simulink model "Extended_2"  (R2019a)
settings: Solver=VariableStepAuto  StartTime=0.0  StopTime=5  RelTol=1e-3
values from neighbouring files (symbols this model uses):
  g = 9.81    [Data.m]    (also in func.m; myTransitionFcn.m)
  m = 0.1    [Data.m]    (also in myTransitionFcn.m)
  r = 0.1    [Data.m]    (also in func.m; myTransitionFcn.m)
  R = 1    [Data.m]    (also in func.m; myTransitionFcn.m)
libraries: simulink x3
settings Model: Creator=Dell  LastModifiedBy=Dell

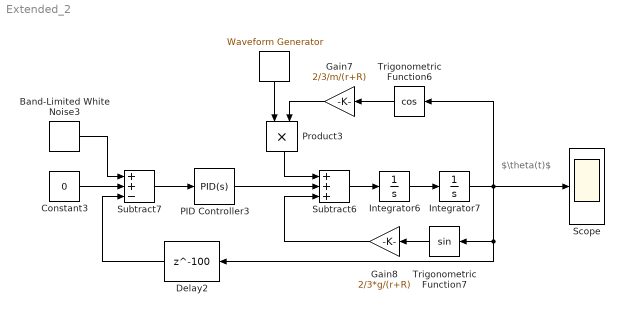
== system Extended_2 ==
  note: $\theta(t)$
  " " : simulink/Sources/Waveform Generator  OutMin=[]  OutMax=[]  OutDataTypeStr=double  SelectedSignal=1  Signals=step()  BlockNames=MultiportSwitch_8c7b78d12e5b405  SampleTime=0.1
      settings: SourceProductName=Simulink
  Band-Limited White Noise3 : simulink/Sources/Band-Limited White Noise  Cov=[0.0001]  Ts=0.1  seed=[23341]
  Constant3 : Constant  Value=0
  Delay2 : Delay  DelayLength=100  InitialCondition=0  UseCircularBuffer=on
  Gain7 : Gain  Gain=2/3/m/(r+R)
  Gain8 : Gain  Gain=2/3*g/(r+R)
  Integrator6 : Integrator
  Integrator7 : Integrator
  PID Controller3 : simulink/Continuous/PID Controller  Controller=PID  Form=Parallel  TimeDomain=Continuous-time  SampleTime=-1  IntegratorMethod=Forward Euler  FilterMethod=Forward Euler  ControllerParametersSource=internal  P=11  I=10  D=6  UseFilter=on  N=141.793807285204  TunerSelectOption=Transfer Function Based (PID Tuner App)  InitialConditionSource=internal  InitialConditionForIntegrator=0  InitialConditionForFilter=0  DifferentiatorICPrevScaledInput=0  ExternalReset=none  TrackingMode=off  Kt=1  LimitOutput=off  UpperSaturationLimit=inf  LowerSaturationLimit=-inf  LinearizeAsGain=on  AntiWindupMode=none  Kb=1  POutMin=[]  POutMax=[]  IOutMin=[]  IOutMax=[]  DOutMin=[]  DOutMax=[]  NOutMin=[]  NOutMax=[]  SumOutMin=[]  SumOutMax=[]  SaturationOutMin=[]  SaturationOutMax=[]  PParamMin=[]  PParamMax=[]  IParamMin=[]  IParamMax=[]  DParamMin=[]  DParamMax=[]  NParamMin=[]  NParamMax=[]  KbParamMin=[]  KbParamMax=[]  KtParamMin=[]  KtParamMax=[]  KbOutMin=[]  KbOutMax=[]  KtOutMin=[]  KtOutMax=[]  IntegratorOutMin=[]  IntegratorOutMax=[]  FilterOutMin=[]  FilterOutMax=[]  SumI1OutMin=[]  SumI1OutMax=[]  SumI2OutMin=[]  SumI2OutMax=[]  SumI3OutMin=[]  SumI3OutMax=[]  SumI4OutMin=[]  SumI4OutMax=[]  SumDOutMin=[]  SumDOutMax=[]  DifferentiatorOutMin=[]  DifferentiatorOutMax=[]  FilterDiffOutCoefMin=[]  FilterDiffOutCoefMax=[]  ReciprocalOutMin=[]  ReciprocalOutMax=[]  SumDenOutMin=[]  SumDenOutMax=[]  SumNumOutMin=[]  SumNumOutMax=[]  DivideOutMin=[]  DivideOutMax=[]  IntegratorContinuousStateAttributes=''  IntegratorStateMustResolveToSignalObject=off  IntegratorRTWStateStorageClass=Auto  FilterContinuousStateAttributes=''  FilterStateMustResolveToSignalObject=off  FilterRTWStateStorageClass=Auto  ParallelPVariant=InternalParameters  IdealPVariant=Disabled  IVariant=InternalParameters  DVariant=InternalParameters  IntegratorVariant=Continuous  SatVariant=Disabled  AWVariant=Passthrough  PCopyVariant=Disabled  TRVariant=Disabled  FdbkBlocksVariant=Forward  IdealPFdbkVariant=Disabled  SatFdbkVariant=Disabled  DerivativeFilterVariant=ContFilter  NVariant=InternalParameters  NCopyVariant=Disabled  FilterICVariant=InternalICsFilter  IntegratorICVariant=InternalICs  ExternalResetVariant=Disabled  TRSumVariant=Passthrough  SumFdbkVariant=Disabled  SumVariant=Sum_PID
  Product3 : Product
  Scope : Scope
  Subtract6 : Sum  Inputs=+++
  Subtract7 : Sum  Inputs=++-
  Trigonometric Function6 : Trigonometry  Operator=cos
  Trigonometric Function7 : Trigonometry
  wires:
  Subtract7/1 -> PID Controller3/1
  Gain8/1 -> Subtract6/3
  " "/1 -> Product3/1
  Trigonometric Function6/1 -> Gain7/1
  Gain7/1 -> Product3/2
  Product3/1 -> Subtract6/1
  Subtract6/1 -> Integrator6/1
  Delay2/1 -> Subtract7/3
  Constant3/1 -> Subtract7/2
  Trigonometric Function7/1 -> Gain8/1
  PID Controller3/1 -> Subtract6/2
  Integrator7/1 -> Trigonometric Function6/1, Scope/1, Trigonometric Function7/1, Delay2/1
  Band-Limited White Noise3/1 -> Subtract7/1
  Integrator6/1 -> Integrator7/1
